simulink model "VVI"  (R2022a)
settings: Solver=FixedStepAuto  StartTime=0.0  StopTime=inf  FixedStep=1e-3  RelTol=1e-3  EnableMultiTasking=on
undefined symbols (not defined in the file): D1, D10, D11, D12, D13, D2, D3, D4, D5, D7, D8, D9, PTA0, PTA1, PTA2, PTB23, PTB9, PTC17, PTC3, PTC4, PTD0, PTD1, PTD2, PTD3
libraries: frdmk64flib x13
settings Model: ExtModeTrigDuration=5  Creator=ethan  LastModifiedBy=gurle
settings OptimizationCC: EnhancedBackFolding=on  PassReuseOutputArgsAs=Individual arguments  ZeroExternalMemoryAtStartup=off  ZeroInternalMemoryAtStartup=off  MaxStackSize=64  OptimizeBlockOrder=speed  DifferentSizesBufferReuse=on  OptimizationCustomize=off  EfficientTunableParamExpr=on
settings DebuggingCC: ParameterTunabilityLossMsg=error
settings HardwareCC: ProdBitPerPointer=32  ProdBitPerSizeT=32  ProdBitPerPtrDiffT=32  ProdLargestAtomicInteger=Long  ProdLargestAtomicFloat=Double  ProdWordSize=32  ProdHWDeviceType=ARM Compatible->ARM Cortex
settings SFSimCC: MATLABDynamicMemAlloc=off
settings RTWCC: SystemTargetFile=ert.tlc  HardwareBoard=NXP FRDM-K64F  TLCOptions="-aInlineSetEventsForThisBaseRateFcn=TLC_FALSE -aSuppressMultiTaskScheduler=TLC_FALSE  -aRateBasedStepFcn=0"  TemplateMakefile=ert_default_tmf  Toolchain=GNU Tools for ARM Embedded Processors
settings CodeAppCC: ForceParamTrailComments=on  IgnoreCustomStorageClasses=off  OperatorAnnotations=on  SimulinkDataObjDesc=on  SFDataObjDesc=on  InsertBlockDesc=on
settings ERTTargetCC: ExtModeTransport=4  ExtModeMexFile=sendToCommService

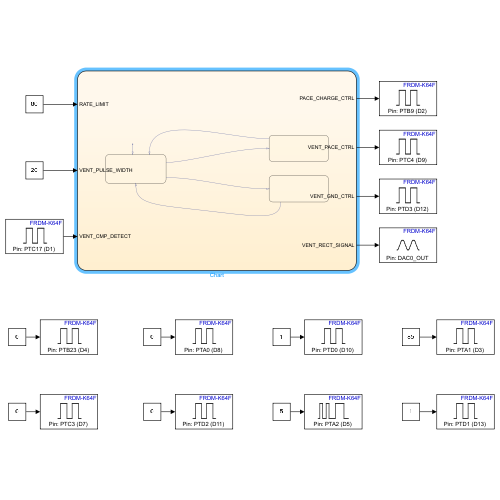
[thumbnail: Simulink's stored preview of the top-level diagram]
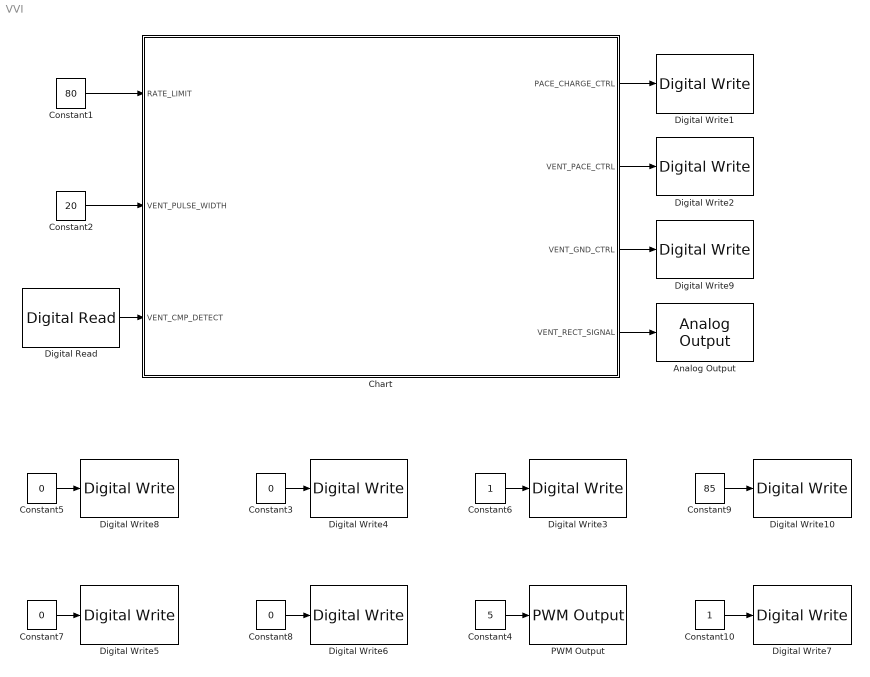
== system VVI ==
  Analog Output : frdmk64flib/Analog Output
      settings: SourceProductBaseCode=EC_FRDM_K64F
  Chart : Stateflow chart  TreatAsAtomicUnit=on
      settings: PortSchema="{\"entries\":[{\"content\":{\"sides\":[{\"content\":{\"connectorIds\":[\"In2\",\"In1\",\"In3\"]},\"type\":\"ConnectorPlacement.EquallySpacedRectSide\",\"uuid\":\"114f396b-5fb5-4ef8-9c98-40ac3a1e57e3\"},{\"content\":{\"connectorIds\":[\"Out1\",\"Out2\",\"Out3\",\"Out4\"],\"side\":\"RIGHT\"},\"type\":\"ConnectorPlacement.EquallySpacedRectSide\",\"uuid\":\"6406f915-9b3f-4d1d-98ef-5d197d381981\"},{\"content\":{\"connectorIds\":[],\"side\":\"TOP\"},\"type\":\"ConnectorPlacement.EquallySpacedRectSide\",\"uuid\":\"d0d8f4a2-d3bb-4a94-b512-bb52efb37fd4\"}]},\"type\":\"ConnectorPlacement.EquallySpacedConnector\",\"uuid\":\"5ab96904-649e-44b7-8e1e-35703c64a9f3\"}],\"packageUris\":[\"http://schema.mathworks.com/mf0/Connector/R2020b\"],\"version\":\"1.0\"}"
  Constant1 : Constant  Value=80  OutDataTypeStr=double
  Constant10 : Constant
  Constant2 : Constant  Value=20
  Constant{3,5,7..8} (4 alike) : Constant  Value=0
  Constant4 : Constant  Value=5
  Constant6 : Constant
  Constant9 : Constant  Value=85
  Digital Read : frdmk64flib/Digital Read  Whichpin=PTC17 (D1)  SampleTime=-1
  Digital Write1 : frdmk64flib/Digital Write  Whichpin=PTB9 (D2)
  Digital Write10 : frdmk64flib/Digital Write  Whichpin=PTA1 (D3)
  Digital Write2 : frdmk64flib/Digital Write  Whichpin=PTC4 (D9)
  Digital Write3 : frdmk64flib/Digital Write  Whichpin=PTD0 (D10)
  Digital Write4 : frdmk64flib/Digital Write  Whichpin=PTA0 (D8)
  Digital Write5 : frdmk64flib/Digital Write  Whichpin=PTC3 (D7)
  Digital Write6 : frdmk64flib/Digital Write  Whichpin=PTD2 (D11)
  Digital Write7 : frdmk64flib/Digital Write  Whichpin=PTD1 (D13)
  Digital Write8 : frdmk64flib/Digital Write  Whichpin=PTB23 (D4)
  Digital Write9 : frdmk64flib/Digital Write  Whichpin=PTD3 (D12)
  PWM Output : frdmk64flib/PWM Output  Whichpin=PTA2 (D5)  InitialFrequency=2000  InitialDutyCycle=0
  wires:
  Chart/1(PACE_CHARGE_CTRL) -> Digital Write1/1
  Constant1/1 -> Chart/2(RATE_LIMIT)
  Constant2/1 -> Chart/1(VENT_PULSE_WIDTH)
  Chart/4(VENT_RECT_SIGNAL) -> Analog Output/1
  Chart/2(VENT_PACE_CTRL) -> Digital Write2/1
  Digital Read/1 -> Chart/3(VENT_CMP_DETECT)
  Constant3/1 -> Digital Write4/1
  Constant4/1 -> PWM Output/1
  Constant5/1 -> Digital Write8/1
  Constant6/1 -> Digital Write3/1
  Constant7/1 -> Digital Write5/1
  Constant8/1 -> Digital Write6/1
  Constant9/1 -> Digital Write10/1
  Constant10/1 -> Digital Write7/1
  Chart/3(VENT_GND_CTRL) -> Digital Write9/1

== stateflow chart VVI/Chart ==
  state SENSED
    entry:
    PACE_CHARGE_CTRL = false;
    VENT_GND_CTRL = true;
    VENT_PACE_CTRL = false;
  state CHARGE_C22
    entry:
    PACE_CHARGE_CTRL = true;
    VENT_GND_CTRL = true;
    VENT_PACE_CTRL = false;
    PACING_REF_PWM = 2000;
  state AV_PACING
    entry:
    PACE_CHARGE_CTRL = false;
    VENT_GND_CTRL = false;
    VENT_PACE_CTRL = true;
  SENSED -> CHARGE_C22 : after((60000/RATE_LIMIT) - VENT_PULSE_WIDTH,msec)
  (default) -> CHARGE_C22
  CHARGE_C22 -> SENSED [order 2] : [VENT_CMP_DETECT == true]
  CHARGE_C22 -> AV_PACING [order 1] : [VENT_CMP_DETECT == false]
  AV_PACING -> CHARGE_C22 : after((60000/RATE_LIMIT) - VENT_PULSE_WIDTH,msec)
  data: PACE_CHARGE_CTRL output; VENT_PACE_CTRL output; VENT_GND_CTRL output; VENT_PULSE_WIDTH input; RATE_LIMIT input; VENT_RECT_SIGNAL output; VENT_CMP_DETECT input
